simulink model "Circle"  (R2016b)
settings: Solver=VariableStepAuto  StartTime=0.0  StopTime=60.0  RelTol=1e-3
settings Model: Creator=Roozbeh  LastModifiedBy=Roozbeh

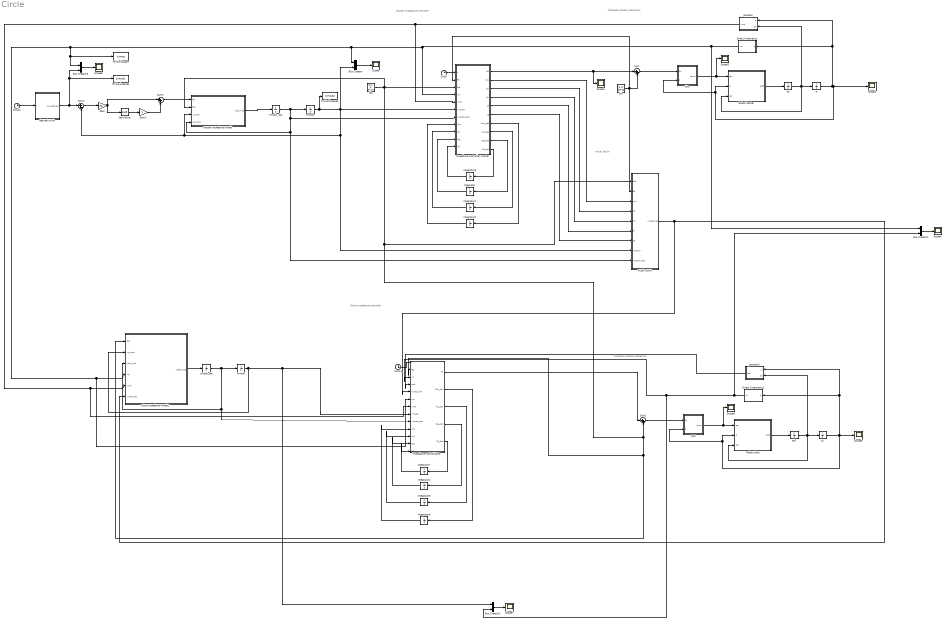
== system Circle ==
  note: Master Impedance controller
  note: Therapist-Master Interaction
  note: Therapist-Master Interaction
  note: Accel. Estim.
  note: Slave Impedance controller
  Accel. Estim. : MATLAB Function  TreatAsAtomicUnit=on
  Bus Creator{,1..3} (4 alike) : BusCreator  Inputs=2
  Clock : Clock
  Clock1 : Clock
  Clock2 : Clock
  Derivative : Derivative
  Direct Kinematics : MATLAB Function  TreatAsAtomicUnit=on
  Direct Kinematics1 : MATLAB Function  TreatAsAtomicUnit=on
  Gain : Gain  Gain=50
  Gain1 : Gain
  Impedance control Slave : MATLAB Function  TreatAsAtomicUnit=on
  Impedance controller master : MATLAB Function  TreatAsAtomicUnit=on
  Integrator{,3..4,7} (4 alike) : Integrator  InitialCondition=rand(3,1*3)'
  Integrator{1..2,5..6} (4 alike) : Integrator  InitialCondition=rand(3,3*3)'
  JTm : MATLAB Function  TreatAsAtomicUnit=on
  JTs1 : MATLAB Function  TreatAsAtomicUnit=on
  Jacobian : MATLAB Function  TreatAsAtomicUnit=on
  Jacobian1 : MATLAB Function  TreatAsAtomicUnit=on
  Master impedance model : MATLAB Function  TreatAsAtomicUnit=on
  Robot Master : MATLAB Function  TreatAsAtomicUnit=on
  Robot slave : MATLAB Function  TreatAsAtomicUnit=on
  Scope{,1..8} (9 alike) : Scope
  Slave impedance model1 : MATLAB Function  TreatAsAtomicUnit=on
  Sum : Sum  Inputs=|++
  Sum1 : Sum  Inputs=|++
  Sum2 : Sum  Inputs=|+-
  Sum3 : Sum  Inputs=|++
  To Workspace : ToWorkspace  VariableName=simout  SaveFormat=Timeseries  SampleTime=-1
  To Workspace1 : ToWorkspace  VariableName=simout1  SaveFormat=Timeseries  SampleTime=-1
  To Workspace2 : ToWorkspace  VariableName=simout2  SaveFormat=Timeseries  SampleTime=-1
  desired circle : MATLAB Function  TreatAsAtomicUnit=on
  fpa : Constant  Value=[0.1; 0; 0]*10
  fth : Constant  Value=[1; 0; 0]*10
  q : Integrator  InitialCondition=[0; 0; 0]
  q1 : Integrator  InitialCondition=[0; 0; 0]
  qd : Integrator  InitialCondition=[0; 0; 0]
  qd1 : Integrator  InitialCondition=[0; 0; 0]
  xmodm : Integrator  InitialCondition=ones(3,1)*5
  xmodm_dot : Integrator  InitialCondition=zeros(3,1)
  xmods : Integrator  InitialCondition=ones(3,1)*5
  xmods_dot : Integrator  InitialCondition=zeros(3,1)
  wires:
  Robot Master/1(qdd) -> qd/1
  qd/1 -> Jacobian/2(qd), q/1, Robot Master/3(qd)
  q/1 -> Scope2/1, JTm/2(q), Robot Master/2(q), Jacobian/1(q), Direct Kinematics/1(q)
  Clock/1 -> Impedance controller master/1(t)
  Impedance controller master/9(Wg_dot) -> Integrator/1
  Integrator/1 -> Impedance controller master/10(Wg)
  Impedance controller master/8(Wc_dot) -> Integrator1/1
  Integrator1/1 -> Impedance controller master/9(Wc)
  Impedance controller master/7(Wm_dot) -> Integrator2/1
  Integrator2/1 -> Impedance controller master/8(Wm)
  Sum/1 -> JTm/1(fm)
  Direct Kinematics/1(xm) -> Bus Creator1/1, To Workspace/1, Bus Creator3/1, Impedance control Slave/6(xm), Slave impedance model1/4(xm), Bus Creator/1, Impedance controller master/4(xm)
  Jacobian/1(xmd) -> Impedance control Slave/7(xmd), Slave impedance model1/5(xmd), Impedance controller master/5(xmd)
  Integrator3/1 -> Impedance controller master/11(Wf)
  Impedance controller master/10(Wf_dot) -> Integrator3/1
  Bus Creator/1 -> Scope/1
  Impedance controller master/1(fm) -> Scope1/1, Sum/1
  Master impedance model/1(xdd_mod) -> xmodm_dot/1
  xmodm_dot/1 -> Accel. Estim./9(xmodm_dot), Master impedance model/4(xd_mod), Impedance controller master/7(xmodm_dot), xmodm/1
  xmodm/1 -> To Workspace2/1, Accel. Estim./8(xmodm), Sum2/2, Master impedance model/3(x_mod), Bus Creator/2, Impedance controller master/6(xmodm)
  fth/1 -> Accel. Estim./2(fth), Sum/2, Impedance controller master/2(fth)
  JTm/1(taum) -> Scope3/1, Robot Master/1(tau)
  Robot slave/1(qdd) -> qd1/1
  qd1/1 -> Robot slave/3(qd), q1/1, Jacobian1/2(qd)
  q1/1 -> Robot slave/2(q), JTs1/2(q), Scope5/1, Direct Kinematics1/1(q), Jacobian1/1(q)
  Sum1/1 -> JTs1/1(fm)
  fpa/1 -> Impedance control Slave/2(fpa), Slave impedance model1/1(fpa), Sum1/2, Accel. Estim./1(fpa), Master impedance model/2(fpa), Impedance controller master/3(fpa)
  JTs1/1(taum) -> Robot slave/1(tau), Scope6/1
  Impedance controller master/2(mm) -> Accel. Estim./3(mm)
  Impedance controller master/3(cm) -> Accel. Estim./4(cm)
  Impedance controller master/4(km) -> Accel. Estim./5(km)
  Impedance controller master/5(kf) -> Accel. Estim./6(kf)
  Impedance controller master/6(x0) -> Accel. Estim./7(x0)
  Slave impedance model1/1(xsdd_mod) -> xmods_dot/1
  xmods_dot/1 -> xmods/1, Impedance control Slave/9(xmods_dot), Slave impedance model1/3(xsd_mod)
  Clock1/1 -> Impedance control Slave/1(t)
  Impedance control Slave/4(Wg_dot) -> Integrator4/1
  Integrator4/1 -> Impedance control Slave/12(Wg)
  Impedance control Slave/3(Wc_dot) -> Integrator5/1
  Integrator5/1 -> Impedance control Slave/11(Wc)
  Impedance control Slave/2(Wm_dot) -> Integrator6/1
  Integrator6/1 -> Impedance control Slave/10(Wm)
  Integrator7/1 -> Impedance control Slave/13(Wf)
  Impedance control Slave/5(Wf_dot) -> Integrator7/1
  Accel. Estim./1(xmdd_hat) -> Impedance control Slave/5(xmdd_hat), Slave impedance model1/6(xmdd_hat)
  Direct Kinematics1/1(xs) -> Bus Creator1/2, Bus Creator2/2, Impedance control Slave/3(xs)
  Jacobian1/1(xsd) -> Impedance control Slave/4(xsd)
  Impedance control Slave/1(fs) -> Sum1/1
  Bus Creator1/1 -> Scope4/1
  xmods/1 -> Bus Creator2/1, Impedance control Slave/8(xmods), Slave impedance model1/2(xs_mod)
  Bus Creator2/1 -> Scope7/1
  Clock2/1 -> desired circle/1(t)
  desired circle/1(Xm_desired) -> To Workspace1/1, Bus Creator3/2, Sum2/1
  Sum2/1 -> Gain/1
  Sum3/1 -> Master impedance model/1(fth)
  Gain/1 -> Derivative/1, Sum3/1
  Derivative/1 -> Gain1/1
  Gain1/1 -> Sum3/2
  Bus Creator3/1 -> Scope8/1

== matlab function Circle/Impedance controller master ==
  data: t input; fth input; fpa input; xm input; xmd input; xmodm input; xmodm_dot input; Wm input; fm output; mm output; cm output; km output; kf output; x0 output; Wc input; Wg input; Wm_dot output; Wc_dot output; Wg_dot output; Wf_dot output; Wf input
function [fm, mm, cm, km, kf, x0, Wm_dot, Wc_dot, Wg_dot, Wf_dot] = fcn(t, fth, fpa, xm, xmd, xmodm, xmodm_dot, Wm, Wc, Wg, Wf)

kf = 1;

fn = 50;
zz = [1; sin(fn*t); sin(2*fn*t)];

Zm = blkdiag(zz,zz,zz);
Zc = Zm;
Zg = zz;
Zf = Zg;

M_hat = Wm' * Zm;
C_hat = Wc' * Zc;
G_hat = Wg' * Zg;
F_hat = Wf' * Zf;

Qm = 100*eye(3*3); %n*l
Qc = 100*eye(3*3);
Qg = 100*eye(1*3);
Qf = 100*eye(1*3);

lambda1m = 1;
lambda2m = 3;
lambda3m = 0;
%a = lambda1m - 1i*lambda3m;
%b = lambda2m + 1i*lambda3m;
%mm = 0.1*eye(3);
% cm = (a+b)*mm*eye(3);
% km = a*b*mm*eye(3);
%cm = 4*mm*eye(3);
%km = 3*mm*eye(3);
mm = 0.75*eye(3);
cm = 2.1*eye(3);
km = 3*eye(3);

xm_tilda = xm - xmodm;
xrm_dot = xmodm_dot - lambda1m*xm_tilda;
x0 = zeros(3,1);
Rm = -(pinv(mm)*cm)*xmd - (pinv(mm)*km)*(xm-x0) + pinv(mm)*(fth-kf*fpa) + lambda3m^2 * xm_tilda;

fm = M_hat* Rm + C_hat*xrm_dot + G_hat + F_hat - fth;


% update
xm_tilda_dot = xmd - xmodm_dot;
sm = xm_tilda_dot + lambda1m*xm_tilda;

Wm_dot = -pinv(Qm)*Zm*Rm*transpose(sm);
Wc_dot = -pinv(Qc)*Zc*xrm_dot*transpose(sm);
Wg_dot = -pinv(Qg)*Zg*transpose(sm);
Wf_dot = -pinv(Qf)*Zf*transpose(sm);

== matlab function Circle/JTm ==
  data: fm input; taum output; q input
function taum = fcn(fm, q)

theta1 = q(1);
theta2 = q(2);
theta3 = q(3);

J11 = 10*sin(theta1)*(38*cos(theta2)*sin(theta3) + 38*sin(theta2)*cos(theta3) + 36*sin(theta2) - 7);
J12 = (-380*cos(theta3) - 360)*cos(theta1)*cos(theta2) + 380*cos(theta1)*sin(theta2)*sin(theta3);
J13 = -380*cos(theta1)*(cos(theta2)*cos(theta3) - sin(theta2)*sin(theta3));
J21 = -10*cos(theta1)*(38*cos(theta2)*sin(theta3) + 38*sin(theta2)*cos(theta3) + 36*sin(theta2) - 7);
J22 = -20*sin(theta1)*(19*cos(theta2)*cos(theta3) - 19*sin(theta2)*sin(theta3) + 18*cos(theta2));
J23 = -380*sin(theta1)*(cos(theta2)*cos(theta3) - sin(theta2)*sin(theta3));
J31 = 0;
J32 = (-380*cos(theta3) - 360)*sin(theta2) - 380*cos(theta2)*sin(theta3);
J33 = -380*cos(theta2)*sin(theta3) - 380*sin(theta2)*cos(theta3);

J = [J11 J12 J13; J21 J22 J23; J31 J32 J33];

taum = J'*fm;

== matlab function Circle/Robot Master ==
  data: tau input; q input; qd input; qdd output
function qdd = fcn(tau, q, qd)

g = 9.81;

theta1 = q(1);
theta2 = q(2);
theta3 = q(3);
qd1 = qd(1);
qd2 = qd(2);
qd3 = qd(3);

G1 = 0;
G2 = -(9*g*(803*cos(theta2)*cos(theta3) - 803*sin(theta2)*sin(theta3) + 4728*sin(theta2)))/10000;
G3 = -(7227*g*(cos(theta2)*cos(theta3) - sin(theta2)*sin(theta3)))/10000;
D11 = ((1300860*cos(theta3)^2 + 5203440*sin(theta3) - 13513230)*cos(theta2)^2)/10000000 - 65043*(7/9 + (sin(theta3) - 4)*sin(theta2))*cos(theta3)*cos(theta2)/500000 - (65043*cos(theta3)^2)/1000000 + ((1011780*sin(theta3) - 5957280)*sin(theta2))/10000000 - (65043*sin(theta3))/125000 + 14294407/10000000;
D12 = 0;
D13 = 0;
D22 = 1351323/1000000 - (65043*sin(theta3))/125000;
D23 = -(65043*sin(theta3))/250000 + 65043/1000000;
D33 = 65043/1000000;
V1 = -(65043*qd1*(cos(theta3)*((qd2 + qd3)*sin(theta3) - 4*qd2 - 2*qd3)*cos(theta2)^2 + (sin(theta2)*(qd2 + qd3)*cos(theta3)^2 + ((4*qd2 + 2*qd3)*sin(theta3) - (16683*qd2)/1606 - qd3/2)*sin(theta2) + (-(7*qd2)/18 - (7*qd3)/18)*sin(theta3) + (5516*qd2)/2409)*cos(theta2) - (7*cos(theta3)*(sin(theta2) + (9*sin(theta3))/7 - 36/7)*(qd2 + qd3))/18))/250000;
V2 = (65043*qd1^2*cos(theta3)^2*cos(theta2)*sin(theta2))/500000 + ((130086*qd1^2*(sin(theta3) - 4)*cos(theta2)^2 - 50589*qd1^2*sin(theta2) - 65043*qd1^2*sin(theta3) + 260172*qd1^2 - 520344*qd3*(qd2 + qd3/2))*cos(theta3))/1000000 + 65043*((sin(theta3) - 16683/6424)*sin(theta2) - (7*sin(theta3))/72 + 1379/2409)*qd1^2*cos(theta2)/125000;
V3 = 65043*(cos(theta3)*(sin(theta3) - 2)*cos(theta2)^2 + (cos(theta3)^2*sin(theta2) + (2*sin(theta3) - 1/2)*sin(theta2) - (7*sin(theta3))/18)*cos(theta2) - 7*(sin(theta2) + (9*sin(theta3))/7 - 36/7)*cos(theta3)/18)*qd1^2/500000 + (65043*qd2^2*cos(theta3))/250000;

G = [G1; G2; G3];
D = [D11 D12 D13; D12 D22 D23; D13 D23 D33];
V = [V1; V2; V3];
F = [qd1; qd2; qd3]*0.05;

qdd = pinv(D)*(tau - V - G - F);

== matlab function Circle/Direct Kinematics ==
  data: q input; xm output
function xm = fcn(q)

theta1 = q(1);
theta2 = q(2);
theta3 = q(3);

xm = [-380*cos(theta1)*(cos(theta2)*sin(theta3) + sin(theta2)*cos(theta3)) + (-360*sin(theta2) + 70)*cos(theta1); ...
    -380*sin(theta1)*(cos(theta2)*sin(theta3) + sin(theta2)*cos(theta3)) + (-360*sin(theta2) + 70)*sin(theta1); ...
    380*cos(theta2)*cos(theta3) - 380*sin(theta2)*sin(theta3) + 360*cos(theta2)];

== matlab function Circle/Jacobian ==
  data: q input; xmd output; qd input
function xmd = fcn(q, qd)

theta1 = q(1);
theta2 = q(2);
theta3 = q(3);

J11 = 10*sin(theta1)*(38*cos(theta2)*sin(theta3) + 38*sin(theta2)*cos(theta3) + 36*sin(theta2) - 7);
J12 = (-380*cos(theta3) - 360)*cos(theta1)*cos(theta2) + 380*cos(theta1)*sin(theta2)*sin(theta3);
J13 = -380*cos(theta1)*(cos(theta2)*cos(theta3) - sin(theta2)*sin(theta3));
J21 = -10*cos(theta1)*(38*cos(theta2)*sin(theta3) + 38*sin(theta2)*cos(theta3) + 36*sin(theta2) - 7);
J22 = -20*sin(theta1)*(19*cos(theta2)*cos(theta3) - 19*sin(theta2)*sin(theta3) + 18*cos(theta2));
J23 = -380*sin(theta1)*(cos(theta2)*cos(theta3) - sin(theta2)*sin(theta3));
J31 = 0;
J32 = (-380*cos(theta3) - 360)*sin(theta2) - 380*cos(theta2)*sin(theta3);
J33 = -380*cos(theta2)*sin(theta3) - 380*sin(theta2)*cos(theta3);

J = [J11 J12 J13; J21 J22 J23; J31 J32 J33];

xmd = J*qd;

== matlab function Circle/Direct Kinematics1 ==
  data: q input; xs output
function xs = fcn(q)

theta1 = q(1);
theta2 = q(2);
theta3 = q(3);

xs = [-380*cos(theta1)*(cos(theta2)*sin(theta3) + sin(theta2)*cos(theta3)) + (-360*sin(theta2) + 70)*cos(theta1); ...
    -380*sin(theta1)*(cos(theta2)*sin(theta3) + sin(theta2)*cos(theta3)) + (-360*sin(theta2) + 70)*sin(theta1); ...
    380*cos(theta2)*cos(theta3) - 380*sin(theta2)*sin(theta3) + 360*cos(theta2)];

== matlab function Circle/Master impedance model ==
  data: fth input; xdd_mod output; fpa input; x_mod input; xd_mod input
function xdd_mod = fcn(fth, fpa, x_mod, xd_mod)

kf = 2;
mm = 0.75*eye(3);
cm = 2.1*eye(3);
km = 3*eye(3);


xdd_mod = pinv(mm)*(fth - kf*fpa - cm*xd_mod - km*x_mod);

end

== matlab function Circle/JTs1 ==
  data: fm input; taum output; q input
function taum = fcn(fm, q)

theta1 = q(1);
theta2 = q(2);
theta3 = q(3);

J11 = 10*sin(theta1)*(38*cos(theta2)*sin(theta3) + 38*sin(theta2)*cos(theta3) + 36*sin(theta2) - 7);
J12 = (-380*cos(theta3) - 360)*cos(theta1)*cos(theta2) + 380*cos(theta1)*sin(theta2)*sin(theta3);
J13 = -380*cos(theta1)*(cos(theta2)*cos(theta3) - sin(theta2)*sin(theta3));
J21 = -10*cos(theta1)*(38*cos(theta2)*sin(theta3) + 38*sin(theta2)*cos(theta3) + 36*sin(theta2) - 7);
J22 = -20*sin(theta1)*(19*cos(theta2)*cos(theta3) - 19*sin(theta2)*sin(theta3) + 18*cos(theta2));
J23 = -380*sin(theta1)*(cos(theta2)*cos(theta3) - sin(theta2)*sin(theta3));
J31 = 0;
J32 = (-380*cos(theta3) - 360)*sin(theta2) - 380*cos(theta2)*sin(theta3);
J33 = -380*cos(theta2)*sin(theta3) - 380*sin(theta2)*cos(theta3);

J = [J11 J12 J13; J21 J22 J23; J31 J32 J33];

taum = J'*fm;

== matlab function Circle/Jacobian1 ==
  data: q input; xsd output; qd input
function xsd = fcn(q, qd)

theta1 = q(1);
theta2 = q(2);
theta3 = q(3);

J11 = 10*sin(theta1)*(38*cos(theta2)*sin(theta3) + 38*sin(theta2)*cos(theta3) + 36*sin(theta2) - 7);
J12 = (-380*cos(theta3) - 360)*cos(theta1)*cos(theta2) + 380*cos(theta1)*sin(theta2)*sin(theta3);
J13 = -380*cos(theta1)*(cos(theta2)*cos(theta3) - sin(theta2)*sin(theta3));
J21 = -10*cos(theta1)*(38*cos(theta2)*sin(theta3) + 38*sin(theta2)*cos(theta3) + 36*sin(theta2) - 7);
J22 = -20*sin(theta1)*(19*cos(theta2)*cos(theta3) - 19*sin(theta2)*sin(theta3) + 18*cos(theta2));
J23 = -380*sin(theta1)*(cos(theta2)*cos(theta3) - sin(theta2)*sin(theta3));
J31 = 0;
J32 = (-380*cos(theta3) - 360)*sin(theta2) - 380*cos(theta2)*sin(theta3);
J33 = -380*cos(theta2)*sin(theta3) - 380*sin(theta2)*cos(theta3);

J = [J11 J12 J13; J21 J22 J23; J31 J32 J33];

xsd = J*qd;

== matlab function Circle/Robot slave ==
  data: tau input; q input; qd input; qdd output
function qdd = fcn(tau, q, qd)

g = 9.81;

theta1 = q(1);
theta2 = q(2);
theta3 = q(3);
qd1 = qd(1);
qd2 = qd(2);
qd3 = qd(3);

G1 = 0;
G2 = -(9*g*(803*cos(theta2)*cos(theta3) - 803*sin(theta2)*sin(theta3) + 4728*sin(theta2)))/10000;
G3 = -(7227*g*(cos(theta2)*cos(theta3) - sin(theta2)*sin(theta3)))/10000;
D11 = ((1300860*cos(theta3)^2 + 5203440*sin(theta3) - 13513230)*cos(theta2)^2)/10000000 - 65043*(7/9 + (sin(theta3) - 4)*sin(theta2))*cos(theta3)*cos(theta2)/500000 - (65043*cos(theta3)^2)/1000000 + ((1011780*sin(theta3) - 5957280)*sin(theta2))/10000000 - (65043*sin(theta3))/125000 + 14294407/10000000;
D12 = 0;
D13 = 0;
D22 = 1351323/1000000 - (65043*sin(theta3))/125000;
D23 = -(65043*sin(theta3))/250000 + 65043/1000000;
D33 = 65043/1000000;
V1 = -(65043*qd1*(cos(theta3)*((qd2 + qd3)*sin(theta3) - 4*qd2 - 2*qd3)*cos(theta2)^2 + (sin(theta2)*(qd2 + qd3)*cos(theta3)^2 + ((4*qd2 + 2*qd3)*sin(theta3) - (16683*qd2)/1606 - qd3/2)*sin(theta2) + (-(7*qd2)/18 - (7*qd3)/18)*sin(theta3) + (5516*qd2)/2409)*cos(theta2) - (7*cos(theta3)*(sin(theta2) + (9*sin(theta3))/7 - 36/7)*(qd2 + qd3))/18))/250000;
V2 = (65043*qd1^2*cos(theta3)^2*cos(theta2)*sin(theta2))/500000 + ((130086*qd1^2*(sin(theta3) - 4)*cos(theta2)^2 - 50589*qd1^2*sin(theta2) - 65043*qd1^2*sin(theta3) + 260172*qd1^2 - 520344*qd3*(qd2 + qd3/2))*cos(theta3))/1000000 + 65043*((sin(theta3) - 16683/6424)*sin(theta2) - (7*sin(theta3))/72 + 1379/2409)*qd1^2*cos(theta2)/125000;
V3 = 65043*(cos(theta3)*(sin(theta3) - 2)*cos(theta2)^2 + (cos(theta3)^2*sin(theta2) + (2*sin(theta3) - 1/2)*sin(theta2) - (7*sin(theta3))/18)*cos(theta2) - 7*(sin(theta2) + (9*sin(theta3))/7 - 36/7)*cos(theta3)/18)*qd1^2/500000 + (65043*qd2^2*cos(theta3))/250000;

G = [G1; G2; G3];
D = [D11 D12 D13; D12 D22 D23; D13 D23 D33];
V = [V1; V2; V3];
F = [qd1; qd2; qd3]*0.05;

qdd = pinv(D)*(tau - V - G - F);

== matlab function Circle/Accel. Estim. ==
  data: fpa input; fth input; mm input; xmdd_hat output; cm input; km input; kf input; x0 input; xmodm input; xmodm_dot input
function xmdd_hat = fcn(fpa, fth, mm, cm, km, kf, x0, xmodm, xmodm_dot)

xmdd_hat = pinv(mm)*(fth-kf*fpa) - pinv(mm)*cm*xmodm_dot - pinv(mm)*km*(xmodm - x0);

== matlab function Circle/Slave impedance model1 ==
  data: xsdd_mod output; fpa input; xs_mod input; xsd_mod input; xm input; xmd input; xmdd_hat input
function xsdd_mod = fcn(fpa, xs_mod, xsd_mod, xm, xmd, xmdd_hat)

kp = 1;
kf = 2;
ms = 25*eye(3);
cs = 3500*eye(3);
ks = 5000*eye(3);

xmods_tilda = xs_mod - kp*xm;
xmods_tilda_dot = xsd_mod - kp*xmd;

xsdd_mod = -pinv(ms)*(fpa +cs*xmods_tilda_dot + ks*xmods_tilda) + xmdd_hat;

end

== matlab function Circle/Impedance control Slave ==
  data: t input; fpa input; xs input; xsd input; xmdd_hat input; xm input; xmd input; xmods input; xmods_dot input; Wm input; fs output; Wc input; Wg input; Wm_dot output; Wc_dot output; Wg_dot output; Wf_dot output; Wf input
function [fs, Wm_dot, Wc_dot, Wg_dot, Wf_dot] = fcn(t, fpa, xs, xsd, xmdd_hat, xm, xmd, ...
    xmods, xmods_dot, Wm, Wc, Wg, Wf)

etha = 1;

kp = 1;
xs_tilda = xs - xmods;
xs_tilda_dot = xsd - xmods_dot;

lambda1s = 4;
lambda2s = lambda1s;
lambda3s = 1;
%a = lambda1m - 1i*lambda3m;
%b = lambda2m + 1i*lambda3m;
ms = 10*eye(3);
% cm = (a+b)*mm*eye(3);
% km = a*b*mm*eye(3);
cs = 8*ms*eye(3);
ks = 17*ms*eye(3);

ss = xs_tilda_dot + lambda1s*xs_tilda;

fn = 50;
zz = [1; sin(fn*t); sin(2*fn*t)];

Zm = blkdiag(zz,zz,zz);
Zc = Zm;
Zg = zz;
Zf = Zg;

M_hat = Wm' * Zm;
C_hat = Wc' * Zc;
G_hat = Wg' * Zg;
F_hat = Wf' * Zf;

Qm = 100*eye(3*3); %n*l
Qc = 100*eye(3*3);
Qg = 100*eye(1*3);
Qf = 100*eye(1*3);

xrs_dot = xmods_dot - lambda1s*xs_tilda;
Rs = kp*xmdd_hat - (pinv(ms)*cs)*(xsd - kp*xmd) - (pinv(ms)*ks)*(xs-kp*xm) - pinv(ms)*(fpa) + lambda3s^2*xs_tilda;

fs = M_hat*Rs + C_hat*xrs_dot + G_hat + F_hat + fpa - etha*sign(ss);

% update
Wm_dot = -pinv(Qm)*Zm*Rs*ss';
Wc_dot = -pinv(Qc)*Zc*xrs_dot*ss';
Wg_dot = -pinv(Qg)*Zg*ss';
Wf_dot = -pinv(Qf)*Zf*ss';

== matlab function Circle/desired circle ==
  data: t input; Xm_desired output
function Xm_desired  = fcn(t)

r = 200; %mm
x = r*sin(2*pi*t/6);
y = r*cos(2*pi*t/6);
z = 300;
Xm_desired = [x; y; z];
